simulink model "RefGenSWD"  (R2018b)
settings: Solver=FixedStepAuto  StartTime=0.0  StopTime=Tsim +Ts*Np  FixedStep=Ts  RelTol=1e-3
values from neighbouring files (symbols this model uses):
  Aref = 10    [simulation.m]    (also in simulationKoop.m)
  fref = 0.5    [simulation.m]    (also in simulationKoop.m)
  Tdref = 0.5    [simulation.m]    (also in simulationKoop.m)
  Tref = 4    [simulation.m]    (also in simulationKoop.m)
  Ts = 0.01    [simulation.m]    (also in simulationKoop.m)
  vehicle = LoadVehicleParameters()    [TransformInputs.m]    (also in mpcController.m; mpcControllerKoop.m; simulation.m; simulationKoop.m)
libraries: simulink_extras x1
settings Model: Creator=Marko  LastModifiedBy=Marko

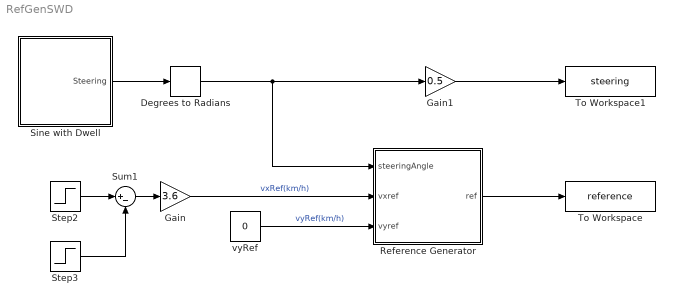
== system RefGenSWD ==
  Degrees to Radians : simulink_extras/Transformations/Degrees to Radians
  Gain : Gain  Gain=3.6
  Gain1 : Gain  Gain=0.5
  Reference Generator : Subsystem
  Sine with Dwell : Subsystem
  Step2 : Step  Time=0  After=80/3.6  SampleTime=0
  Step3 : Step  Time=5  After=0  SampleTime=0
  Sum1 : Sum  Inputs=|+-
  To Workspace : ToWorkspace  VariableName=reference  SaveFormat=Structure With Time  SampleTime=Ts
  To Workspace1 : ToWorkspace  VariableName=steering  SaveFormat=Structure With Time  SampleTime=Ts
  vyRef : Constant  Value=0
  wires:
  Sine with Dwell/1(Steering) -> Degrees to Radians/1
  Sum1/1 -> Gain/1
  Step2/1 -> Sum1/1
  vyRef/1 -> Reference Generator/3(vyref)  "vyRef(km/h)"
  Gain/1 -> Reference Generator/2(vxref)  "vxRef(km/h)"
  Step3/1 -> Sum1/2
  Reference Generator/1(ref) -> To Workspace/1
  Degrees to Radians/1 -> Reference Generator/1(steeringAngle), Gain1/1
  Gain1/1 -> To Workspace1/1

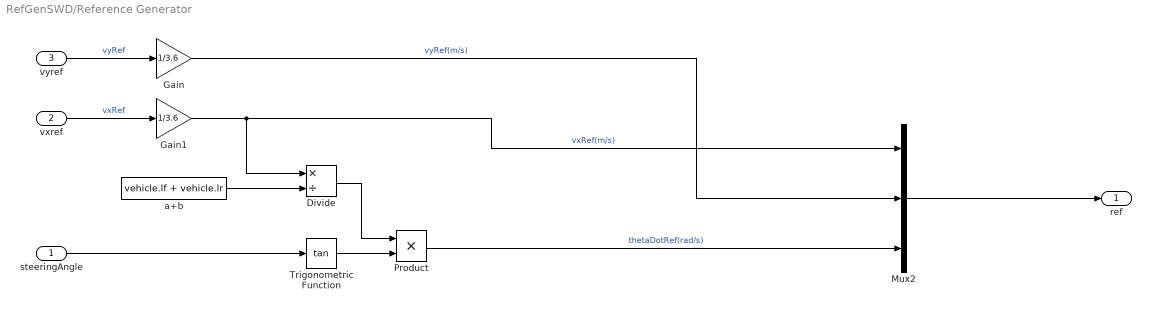
== system RefGenSWD/Reference Generator ==
  steeringAngle : Inport
  vxref : Inport  Port=2
  vyref : Inport  Port=3
  Divide : Product  Inputs=*/
  Gain : Gain  Gain=1/3.6
  Gain1 : Gain  Gain=1/3.6
  Mux2 : Mux  Inputs=3
  Product : Product
  Trigonometric Function : Trigonometry  Operator=tan  OutputSignalType=real
  a+b : Constant  Value=vehicle.lf + vehicle.lr
  ref : Outport
  wires:
  a+b/1 -> Divide/2
  vxref/1 -> Gain1/1  "vxRef"
  Product/1 -> Mux2/3  "thetaDotRef(rad/s)"
  Divide/1 -> Product/1
  Trigonometric Function/1 -> Product/2
  steeringAngle/1 -> Trigonometric Function/1
  Mux2/1 -> ref/1
  vyref/1 -> Gain/1  "vyRef"
  Gain1/1 -> Mux2/1, Divide/1  "vxRef(m/s)"
  Gain/1 -> Mux2/2  "vyRef(m/s)"

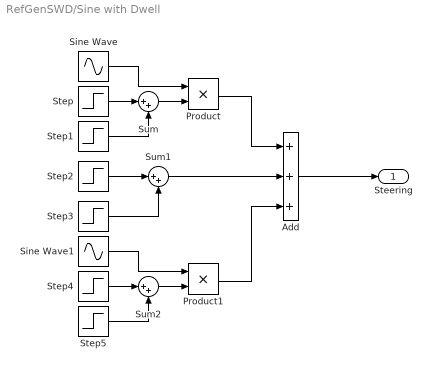
== system RefGenSWD/Sine with Dwell ==
  Add : Sum  Inputs=+++
  Product : Product
  Product1 : Product
  Sine Wave : Sin  Amplitude=Aref  Frequency=2*pi*fref  Phase=-2*pi*fref*Tref  SampleTime=0
  Sine Wave1 : Sin  Amplitude=Aref  Frequency=2*pi*fref  Phase=-2*pi*fref*(Tref+Tdref)  SampleTime=0
  Step : Step  Time=Tref  SampleTime=0
  Step1 : Step  Time=Tref+0.75/fref  After=-1  SampleTime=0
  Step2 : Step  Time=Tref+0.75/fref  After=-Aref  SampleTime=0
  Step3 : Step  Time=Tref+0.75/fref+Tdref  After=Aref  SampleTime=0
  Step4 : Step  Time=Tref+0.75/fref+Tdref  SampleTime=0
  Step5 : Step  Time=Tref+1/fref+Tdref  After=-1  SampleTime=0
  Sum : Sum  Inputs=|++
  Sum1 : Sum  Inputs=|++
  Sum2 : Sum  Inputs=|++
  Steering : Outport
  wires:
  Step2/1 -> Sum1/1
  Sine Wave/1 -> Product/1
  Add/1 -> Steering/1
  Sum1/1 -> Add/2
  Step3/1 -> Sum1/2
  Sum2/1 -> Product1/2
  Product1/1 -> Add/3
  Sine Wave1/1 -> Product1/1
  Step1/1 -> Sum/2
  Step/1 -> Sum/1
  Product/1 -> Add/1
  Step4/1 -> Sum2/1
  Step5/1 -> Sum2/2
  Sum/1 -> Product/2
